simulink model "SlidingModeAdaptiveControl_Example"  (R2019a)
settings: Solver=VariableStepAuto  StartTime=0.0  StopTime=10.0  RelTol=1e-3
settings Model: Creator=0629w  LastModifiedBy=0629w

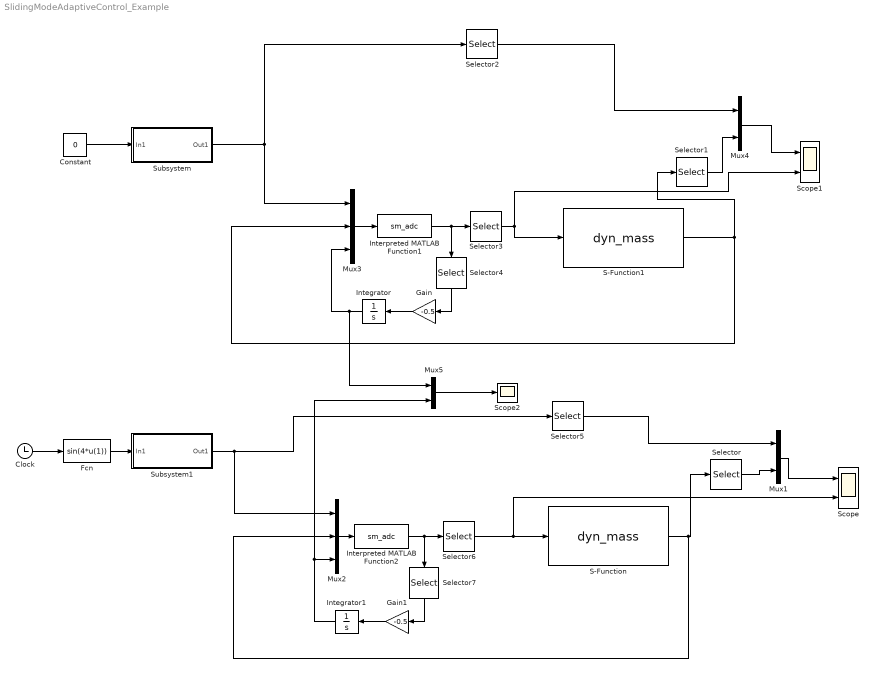
== system SlidingModeAdaptiveControl_Example ==
  Clock : Clock
  Constant : Constant  Value=0
  Fcn : Fcn  Expr=sin(4*u(1))
  Gain : Gain  Gain=-0.5
  Gain1 : Gain  Gain=-0.5
  Integrator : Integrator
  Integrator1 : Integrator
  Interpreted MATLAB Function1 : MATLABFcn  MATLABFcn=sm_adc  OutputDimensions=2
  Interpreted MATLAB Function2 : MATLABFcn  MATLABFcn=sm_adc  OutputDimensions=2
  Mux1 : Mux  Inputs=2
  Mux2 : Mux  Inputs=3
  Mux3 : Mux  Inputs=3
  Mux4 : Mux  Inputs=2
  Mux5 : Mux  Inputs=2
  S-Function : S-Function  FunctionName=dyn_mass  SFunctionDeploymentMode=off  EnableBusSupport=off
  S-Function1 : S-Function  FunctionName=dyn_mass  SFunctionDeploymentMode=off  EnableBusSupport=off
  Scope : Scope  NumInputPorts=2
  Scope1 : Scope  NumInputPorts=2
  Scope2 : Scope
  Selector{,1,3,6} (4 alike) : Selector  InputPortWidth=2  IndexOptions=Index vector (dialog)  Indices=[1]  OutputSizes=1
  Selector2 : Selector  InputPortWidth=3  IndexOptions=Index vector (dialog)  Indices=[1]  OutputSizes=1
  Selector4 : Selector  InputPortWidth=2  IndexOptions=Index vector (dialog)  Indices=[2]  OutputSizes=1
  Selector5 : Selector  InputPortWidth=3  IndexOptions=Index vector (dialog)  Indices=[1]  OutputSizes=1
  Selector7 : Selector  IndexMode=Zero-based  InputPortWidth=2  IndexOptions=Index vector (dialog)  Indices=[1]  OutputSizes=1
  Subsystem : Subsystem
  Subsystem1 : Subsystem
  wires:
  Clock/1 -> Fcn/1
  S-Function/1 -> Mux2/2, Selector/1
  Mux1/1 -> Scope/1
  Selector/1 -> Mux1/2
  Mux4/1 -> Scope1/1
  Selector1/1 -> Mux4/2
  Constant/1 -> Subsystem/1(In1)
  Subsystem/1(Out1) -> Mux3/1, Selector2/1
  Integrator/1 -> Mux5/1, Mux3/3
  Gain/1 -> Integrator/1
  Interpreted MATLAB Function1/1 -> Selector3/1, Selector4/1
  Selector3/1 -> Scope1/2, S-Function1/1
  Selector4/1 -> Gain/1
  S-Function1/1 -> Mux3/2, Selector1/1
  Selector2/1 -> Mux4/1
  Mux3/1 -> Interpreted MATLAB Function1/1
  Mux5/1 -> Scope2/1
  Fcn/1 -> Subsystem1/1(In1)
  Subsystem1/1(Out1) -> Selector5/1, Mux2/1
  Selector5/1 -> Mux1/1
  Gain1/1 -> Integrator1/1
  Mux2/1 -> Interpreted MATLAB Function2/1
  Selector7/1 -> Gain1/1
  Interpreted MATLAB Function2/1 -> Selector6/1, Selector7/1
  Integrator1/1 -> Mux5/2, Mux2/3
  Selector6/1 -> Scope/2, S-Function/1

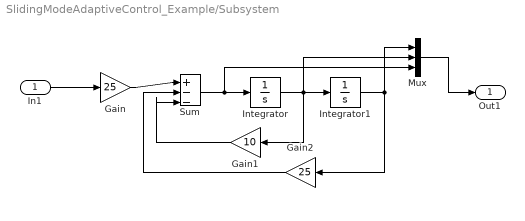
== system SlidingModeAdaptiveControl_Example/Subsystem ==
  In1 : Inport
  Gain : Gain  Gain=25
  Gain1 : Gain  Gain=10
  Gain2 : Gain  Gain=25
  Integrator : Integrator
  Integrator1 : Integrator
  Mux : Mux  Inputs=3
  Sum : Sum  Inputs=|+--
  Out1 : Outport
  wires:
  In1/1 -> Gain/1
  Gain/1 -> Sum/1
  Sum/1 -> Mux/3, Integrator/1
  Integrator/1 -> Mux/2, Integrator1/1, Gain1/1
  Integrator1/1 -> Mux/1, Gain2/1
  Gain1/1 -> Sum/3
  Gain2/1 -> Sum/2
  Mux/1 -> Out1/1

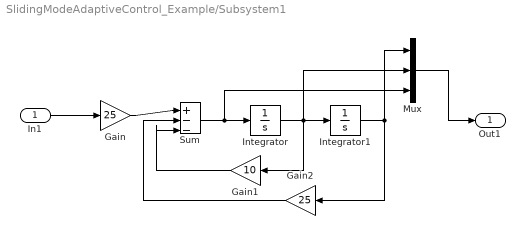
== system SlidingModeAdaptiveControl_Example/Subsystem1 ==
  In1 : Inport
  Gain : Gain  Gain=25
  Gain1 : Gain  Gain=10
  Gain2 : Gain  Gain=25
  Integrator : Integrator
  Integrator1 : Integrator
  Mux : Mux  Inputs=3
  Sum : Sum  Inputs=|+--
  Out1 : Outport
  wires:
  In1/1 -> Gain/1
  Gain/1 -> Sum/1
  Sum/1 -> Mux/3, Integrator/1
  Integrator/1 -> Mux/2, Integrator1/1, Gain1/1
  Integrator1/1 -> Mux/1, Gain2/1
  Gain1/1 -> Sum/3
  Gain2/1 -> Sum/2
  Mux/1 -> Out1/1
